simulink model "LoFT_Example3"  (R2024b)
settings: Solver=ode4  StartTime=0.0  StopTime=300  FixedStep=simu.dt  RelTol=1e-3
undefined symbols (not defined in the file): body, circtime, Communication, D1, Delta, irkb, line, LoFT, p0, Pn, s, simu, trip_time, Turbwind, waves, wind
libraries: simulink x350, spsThreePhaseVIMeasurementLib x41, spsThreePhasePISectionLineLib x34, spsThreePhaseParallelRLCLoadLib x21, spsThreePhaseTransformerTwoWindingsLib x14, spsLoadFlowBusLib x10, spsThreePhaseDynamicLoadLib x9, spsSynchronousMachinepuStandardLib x7, spsExcitationSystemLib x7, spsSteamTurbineandGovernorLib x7, spsGenericPowerSystemStabilizerLib x7, spsMultiBandPowerSystemStabilizerLib x7
(part 2 of 49)

== system LoFT_Example3/FOWT System/Subsystem13 ==
  action : Inport
  In2 : Inport  Port=2
  In1 : Inport  Port=3
  Constant1 : Constant  Value=Communication(5)
  Constant10 : Constant  Value=Communication(3)
  Constant11 : Constant  Value=Communication(9)
  Constant12 : Constant  Value=Communication(6)
  Constant14 : Constant  Value=Communication(7)
  Constant16 : Constant  Value=Communication(8)
  Constant19 : Constant  Value=Communication(10)
  Constant7 : Constant  Value=Communication(4)
  Constant8 : Constant  Value=Communication(1)
  Constant9 : Constant  Value=Communication(2)
  Demux : Demux  Outputs=10
  Demux1 : Demux  Outputs=10
  FOWT1 : Subsystem  mask{Aero=LoFT.Aero, Hydro=LoFT.Hydro, Mooring=LoFT.Mooring, Property=LoFT.Property, Controller=LoFT.Controller, Initposition=[15,  0,  3*pi/180], Initstate=[6.8*pi/30, 9]}
      mask prompts: Aero "Aerodynamics"; Hydro "Hydrodynamics"; Mooring "Mooring lookup table"; Property "Hull mass, inertia and volume"; Controller "Local controller"; Initposition "Initial Hull position"; Initstate "Initial RotSpeed and WindEst"
      mask DialogControl DescGroupVar Prompt: LoFT
      mask DialogControl FOWT Prompt: Low-order modelling of floating offshore wind turbine for training
      mask DialogControl Manuscript Prompt: Citation
      mask DialogControl scriptname Prompt: Primary Frequency Response of Floating Offshore Wind Turbines via Deep Reinforcement Learning and Domain Randomization
      mask DialogControl ParameterGroupVar Prompt: 参数
  FOWT10 : Subsystem  mask{Aero=LoFT.Aero, Hydro=LoFT.Hydro, Mooring=LoFT.Mooring, Property=LoFT.Property, Controller=LoFT.Controller, Initposition=[5,  0,  3*pi/180], Initstate=[6.8*pi/30, 9]}
      mask prompts: Aero "Aerodynamics"; Hydro "Hydrodynamics"; Mooring "Mooring lookup table"; Property "Hull mass, inertia and volume"; Controller "Local controller"; Initposition "Initial Hull position"; Initstate "Initial RotSpeed and WindEst"
      mask DialogControl DescGroupVar Prompt: LoFT
      mask DialogControl FOWT Prompt: Low-order modelling of floating offshore wind turbine for training
      mask DialogControl Manuscript Prompt: Citation
      mask DialogControl scriptname Prompt: Primary Frequency Response of Floating Offshore Wind Turbines via Deep Reinforcement Learning and Domain Randomization
      mask DialogControl ParameterGroupVar Prompt: 参数
  FOWT2 : Subsystem  mask{Aero=LoFT.Aero, Hydro=LoFT.Hydro, Mooring=LoFT.Mooring, Property=LoFT.Property, Controller=LoFT.Controller, Initposition=[40,  0,  3*pi/180], Initstate=[6.8*pi/30, 9]}
      mask prompts: Aero "Aerodynamics"; Hydro "Hydrodynamics"; Mooring "Mooring lookup table"; Property "Hull mass, inertia and volume"; Controller "Local controller"; Initposition "Initial Hull position"; Initstate "Initial RotSpeed and WindEst"
      mask DialogControl DescGroupVar Prompt: LoFT
      mask DialogControl FOWT Prompt: Low-order modelling of floating offshore wind turbine for training
      mask DialogControl Manuscript Prompt: Citation
      mask DialogControl scriptname Prompt: Primary Frequency Response of Floating Offshore Wind Turbines via Deep Reinforcement Learning and Domain Randomization
      mask DialogControl ParameterGroupVar Prompt: 参数
  FOWT3 : Subsystem  mask{Aero=LoFT.Aero, Hydro=LoFT.Hydro, Mooring=LoFT.Mooring, Property=LoFT.Property, Controller=LoFT.Controller, Initposition=[25,  0,  3*pi/180], Initstate=[6.8*pi/30, 9]}
      mask prompts: Aero "Aerodynamics"; Hydro "Hydrodynamics"; Mooring "Mooring lookup table"; Property "Hull mass, inertia and volume"; Controller "Local controller"; Initposition "Initial Hull position"; Initstate "Initial RotSpeed and WindEst"
      mask DialogControl DescGroupVar Prompt: LoFT
      mask DialogControl FOWT Prompt: Low-order modelling of floating offshore wind turbine for training
      mask DialogControl Manuscript Prompt: Citation
      mask DialogControl scriptname Prompt: Primary Frequency Response of Floating Offshore Wind Turbines via Deep Reinforcement Learning and Domain Randomization
      mask DialogControl ParameterGroupVar Prompt: 参数
  FOWT4 : Subsystem  mask{Aero=LoFT.Aero, Hydro=LoFT.Hydro, Mooring=LoFT.Mooring, Property=LoFT.Property, Controller=LoFT.Controller, Initposition=[15,  0,  3*pi/180], Initstate=[6.8*pi/30, 9]}
      mask prompts: Aero "Aerodynamics"; Hydro "Hydrodynamics"; Mooring "Mooring lookup table"; Property "Hull mass, inertia and volume"; Controller "Local controller"; Initposition "Initial Hull position"; Initstate "Initial RotSpeed and WindEst"
      mask DialogControl DescGroupVar Prompt: LoFT
      mask DialogControl FOWT Prompt: Low-order modelling of floating offshore wind turbine for training
      mask DialogControl Manuscript Prompt: Citation
      mask DialogControl scriptname Prompt: Primary Frequency Response of Floating Offshore Wind Turbines via Deep Reinforcement Learning and Domain Randomization
      mask DialogControl ParameterGroupVar Prompt: 参数
  FOWT5 : Subsystem  mask{Aero=LoFT.Aero, Hydro=LoFT.Hydro, Mooring=LoFT.Mooring, Property=LoFT.Property, Controller=LoFT.Controller, Initposition=[40,  0,  3*pi/180], Initstate=[6.8*pi/30, 9]}
      mask prompts: Aero "Aerodynamics"; Hydro "Hydrodynamics"; Mooring "Mooring lookup table"; Property "Hull mass, inertia and volume"; Controller "Local controller"; Initposition "Initial Hull position"; Initstate "Initial RotSpeed and WindEst"
      mask DialogControl DescGroupVar Prompt: LoFT
      mask DialogControl FOWT Prompt: Low-order modelling of floating offshore wind turbine for training
      mask DialogControl Manuscript Prompt: Citation
      mask DialogControl scriptname Prompt: Primary Frequency Response of Floating Offshore Wind Turbines via Deep Reinforcement Learning and Domain Randomization
      mask DialogControl ParameterGroupVar Prompt: 参数
  FOWT6 : Subsystem  mask{Aero=LoFT.Aero, Hydro=LoFT.Hydro, Mooring=LoFT.Mooring, Property=LoFT.Property, Controller=LoFT.Controller, Initposition=[25,  0,  3*pi/180], Initstate=[6.8*pi/30, 9]}
      mask prompts: Aero "Aerodynamics"; Hydro "Hydrodynamics"; Mooring "Mooring lookup table"; Property "Hull mass, inertia and volume"; Controller "Local controller"; Initposition "Initial Hull position"; Initstate "Initial RotSpeed and WindEst"
      mask DialogControl DescGroupVar Prompt: LoFT
      mask DialogControl FOWT Prompt: Low-order modelling of floating offshore wind turbine for training
      mask DialogControl Manuscript Prompt: Citation
      mask DialogControl scriptname Prompt: Primary Frequency Response of Floating Offshore Wind Turbines via Deep Reinforcement Learning and Domain Randomization
      mask DialogControl ParameterGroupVar Prompt: 参数
  FOWT7 : Subsystem  mask{Aero=LoFT.Aero, Hydro=LoFT.Hydro, Mooring=LoFT.Mooring, Property=LoFT.Property, Controller=LoFT.Controller, Initposition=[15,  0,  3*pi/180], Initstate=[6.8*pi/30, 9]}
      mask prompts: Aero "Aerodynamics"; Hydro "Hydrodynamics"; Mooring "Mooring lookup table"; Property "Hull mass, inertia and volume"; Controller "Local controller"; Initposition "Initial Hull position"; Initstate "Initial RotSpeed and WindEst"
      mask DialogControl DescGroupVar Prompt: LoFT
      mask DialogControl FOWT Prompt: Low-order modelling of floating offshore wind turbine for training
      mask DialogControl Manuscript Prompt: Citation
      mask DialogControl scriptname Prompt: Primary Frequency Response of Floating Offshore Wind Turbines via Deep Reinforcement Learning and Domain Randomization
      mask DialogControl ParameterGroupVar Prompt: 参数
  FOWT8 : Subsystem  mask{Aero=LoFT.Aero, Hydro=LoFT.Hydro, Mooring=LoFT.Mooring, Property=LoFT.Property, Controller=LoFT.Controller, Initposition=[40,  0,  3*pi/180], Initstate=[6.8*pi/30, 9]}
      mask prompts: Aero "Aerodynamics"; Hydro "Hydrodynamics"; Mooring "Mooring lookup table"; Property "Hull mass, inertia and volume"; Controller "Local controller"; Initposition "Initial Hull position"; Initstate "Initial RotSpeed and WindEst"
      mask DialogControl DescGroupVar Prompt: LoFT
      mask DialogControl FOWT Prompt: Low-order modelling of floating offshore wind turbine for training
      mask DialogControl Manuscript Prompt: Citation
      mask DialogControl scriptname Prompt: Primary Frequency Response of Floating Offshore Wind Turbines via Deep Reinforcement Learning and Domain Randomization
      mask DialogControl ParameterGroupVar Prompt: 参数
  FOWT9 : Subsystem  mask{Aero=LoFT.Aero, Hydro=LoFT.Hydro, Mooring=LoFT.Mooring, Property=LoFT.Property, Controller=LoFT.Controller, Initposition=[25,  0,  3*pi/180], Initstate=[6.8*pi/30, 9]}
      mask prompts: Aero "Aerodynamics"; Hydro "Hydrodynamics"; Mooring "Mooring lookup table"; Property "Hull mass, inertia and volume"; Controller "Local controller"; Initposition "Initial Hull position"; Initstate "Initial RotSpeed and WindEst"
      mask DialogControl DescGroupVar Prompt: LoFT
      mask DialogControl FOWT Prompt: Low-order modelling of floating offshore wind turbine for training
      mask DialogControl Manuscript Prompt: Citation
      mask DialogControl scriptname Prompt: Primary Frequency Response of Floating Offshore Wind Turbines via Deep Reinforcement Learning and Domain Randomization
      mask DialogControl ParameterGroupVar Prompt: 参数
  "switch " : Subsystem
  switch 1 : Subsystem
  switch 2 : Subsystem
  switch 3 : Subsystem
  switch 4 : Subsystem
  switch 5 : Subsystem
  switch 6 : Subsystem
  switch 7 : Subsystem
  switch 8 : Subsystem
  switch 9 : Subsystem
  wave series 1 : Subsystem
  wave series 10 : Subsystem
  wave series 2 : Subsystem
  wave series 3 : Subsystem
  wave series 4 : Subsystem
  wave series 5 : Subsystem
  wave series 6 : Subsystem
  wave series 7 : Subsystem
  wave series 8 : Subsystem
  wave series 9 : Subsystem
  1 : Outport
  2 : Outport  Port=2
  3 : Outport  Port=3
  4 : Outport  Port=4
  5 : Outport  Port=5
  6 : Outport  Port=6
  7 : Outport  Port=7
  8 : Outport  Port=8
  9 : Outport  Port=9
  10 : Outport  Port=10
  wires:
  [B1] -> FOWT6/4(Blade Pitch(rad))
  [B1] -> FOWT5/4(Blade Pitch(rad))
  [B1] -> FOWT4/4(Blade Pitch(rad))
  [B1] -> FOWT3/4(Blade Pitch(rad))
  [B1] -> FOWT2/4(Blade Pitch(rad))
  [B1] -> FOWT1/4(Blade Pitch(rad))
  In1/1 -> [B1]
  FOWT10/1(Out1) -> 10/1
  FOWT9/1(Out1) -> 9/1
  FOWT8/1(Out1) -> 8/1
  FOWT7/1(Out1) -> 7/1
  FOWT6/1(Out1) -> 6/1
  FOWT5/1(Out1) -> 5/1
  FOWT4/1(Out1) -> 4/1
  FOWT3/1(Out1) -> 3/1
  FOWT2/1(Out1) -> 2/1
  FOWT1/1(Out1) -> 1/1
  Demux1/6 -> [Wind6]
  Demux1/1 -> [Wind1]
  Demux1/10 -> [Wind10]
  Demux1/9 -> [Wind9]
  Demux1/5 -> [Wind5]
  Demux1/2 -> [Wind2]
  Demux1/3 -> [Wind3]
  Demux1/8 -> [Wind8]
  Demux1/7 -> [Wind7]
  In2/1 -> Demux1/1
  Demux1/4 -> [Wind4]
  switch 2/1(Out1) -> FOWT3/5(Commu)
  switch 3/1(Out1) -> FOWT4/5(Commu)
  switch 5/1(Out1) -> FOWT6/5(Commu)
  [P7] -> FOWT7/3(Power(MW))
  Constant9/1 -> switch 1/1(In1)
  Constant7/1 -> switch 3/1(In1)
  wave series 3/1(Out1) -> FOWT3/2(Waveforces)
  [Wind6] -> FOWT6/1(Inflow wind(m/s))
  [P2] -> FOWT2/3(Power(MW))
  [Wind1] -> FOWT1/1(Inflow wind(m/s))
  switch 1/1(Out1) -> FOWT2/5(Commu)
  Constant1/1 -> switch 4/1(In1)
  [P3] -> FOWT3/3(Power(MW))
  [B1] -> FOWT7/4(Blade Pitch(rad))
  [P1] -> FOWT1/3(Power(MW))
  [Wind7] -> FOWT7/1(Inflow wind(m/s))
  wave series 7/1(Out1) -> FOWT7/2(Waveforces)
  [P4] -> FOWT4/3(Power(MW))
  Constant12/1 -> switch 5/1(In1)
  [P6] -> FOWT6/3(Power(MW))
  Constant14/1 -> switch 6/1(In1)
  [P5] -> FOWT5/3(Power(MW))
  Constant10/1 -> switch 2/1(In1)
  wave series 5/1(Out1) -> FOWT5/2(Waveforces)
  [B1] -> FOWT8/4(Blade Pitch(rad))
  [P8] -> FOWT8/3(Power(MW))
  "switch "/1(Out1) -> FOWT1/5(Commu)
  Constant8/1 -> "switch "/1(In1)
  [Wind5] -> FOWT5/1(Inflow wind(m/s))
  wave series 1/1(Out1) -> FOWT1/2(Waveforces)
  [Wind8] -> FOWT8/1(Inflow wind(m/s))
  wave series 6/1(Out1) -> FOWT6/2(Waveforces)
  Constant16/1 -> switch 7/1(In1)
  switch 6/1(Out1) -> FOWT7/5(Commu)
  wave series 4/1(Out1) -> FOWT4/2(Waveforces)
  switch 7/1(Out1) -> FOWT8/5(Commu)
  switch 4/1(Out1) -> FOWT5/5(Commu)
  [Wind3] -> FOWT3/1(Inflow wind(m/s))
  wave series 8/1(Out1) -> FOWT8/2(Waveforces)
  [Wind4] -> FOWT4/1(Inflow wind(m/s))
  wave series 2/1(Out1) -> FOWT2/2(Waveforces)
  [Wind2] -> FOWT2/1(Inflow wind(m/s))
  Demux/2 -> [P2]
  Demux/3 -> [P3]
  action/1 -> Demux/1
  Demux/4 -> [P4]
  Demux/1 -> [P1]
  Demux/5 -> [P5]
  Demux/8 -> [P8]
  Demux/7 -> [P7]
  Demux/6 -> [P6]
  wave series 9/1(Out1) -> FOWT9/2(Waveforces)
  switch 8/1(Out1) -> FOWT9/5(Commu)
  [Wind9] -> FOWT9/1(Inflow wind(m/s))
  [B1] -> FOWT9/4(Blade Pitch(rad))
  [P9] -> FOWT9/3(Power(MW))
  Constant11/1 -> switch 8/1(In1)
  [Wind10] -> FOWT10/1(Inflow wind(m/s))
  [P10] -> FOWT10/3(Power(MW))
  switch 9/1(Out1) -> FOWT10/5(Commu)
  Constant19/1 -> switch 9/1(In1)
  [B1] -> FOWT10/4(Blade Pitch(rad))
  wave series 10/1(Out1) -> FOWT10/2(Waveforces)
  Demux/10 -> [P10]
  Demux/9 -> [P9]

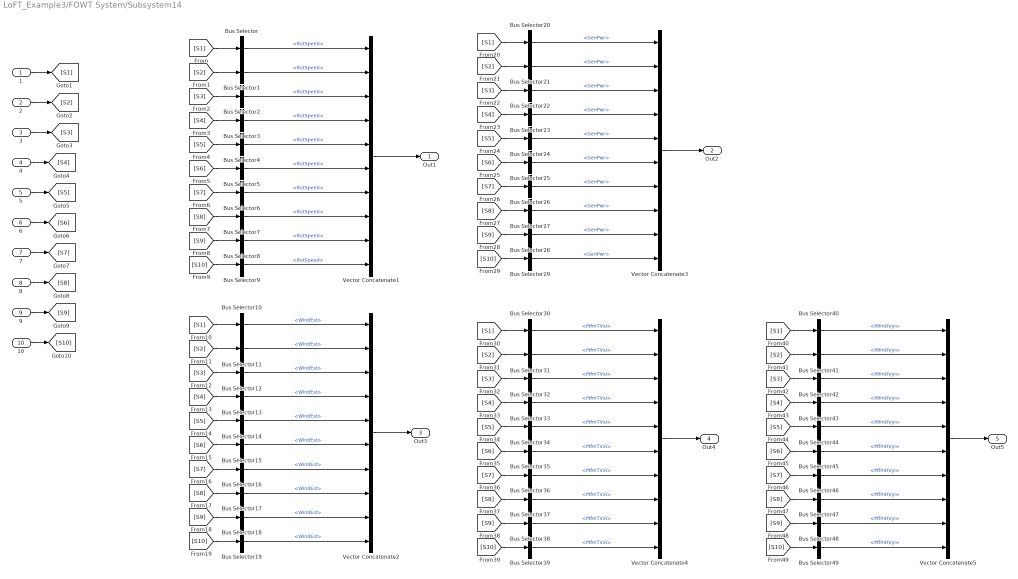
== system LoFT_Example3/FOWT System/Subsystem14 ==
  1 : Inport
  2 : Inport  Port=2
  3 : Inport  Port=3
  4 : Inport  Port=4
  5 : Inport  Port=5
  6 : Inport  Port=6
  7 : Inport  Port=7
  8 : Inport  Port=8
  9 : Inport  Port=9
  10 : Inport  Port=10
  Bus Selector{,1..9} (10 alike) : BusSelector  OutputSignals=RotSpeed
  Bus Selector{10..19} (10 alike) : BusSelector  OutputSignals=WindEst
  Bus Selector{20..29} (10 alike) : BusSelector  OutputSignals=GenPwr
  Bus Selector{30..39} (10 alike) : BusSelector  OutputSignals=PtfmTVxi
  Bus Selector{40..49} (10 alike) : BusSelector  OutputSignals=PtfmRVyi
  Vector Concatenate{1..5} (5 alike) : Concatenate  NumInputs=10
  Out1 : Outport
  Out2 : Outport  Port=2
  Out3 : Outport  Port=3
  Out4 : Outport  Port=4
  Out5 : Outport  Port=5
  wires:
  1/1 -> [S1]
  2/1 -> [S2]
  3/1 -> [S3]
  4/1 -> [S4]
  5/1 -> [S5]
  6/1 -> [S6]
  7/1 -> [S7]
  8/1 -> [S8]
  9/1 -> [S9]
  10/1 -> [S10]
  [S1] -> Bus Selector/1
  Vector Concatenate1/1 -> Out1/1
  Bus Selector/1 -> Vector Concatenate1/1  "<RotSpeed>"
  [S2] -> Bus Selector1/1
  Bus Selector1/1 -> Vector Concatenate1/2  "<RotSpeed>"
  Bus Selector2/1 -> Vector Concatenate1/3  "<RotSpeed>"
  [S3] -> Bus Selector2/1
  [S4] -> Bus Selector3/1
  Bus Selector3/1 -> Vector Concatenate1/4  "<RotSpeed>"
  [S5] -> Bus Selector4/1
  [S6] -> Bus Selector5/1
  [S7] -> Bus Selector6/1
  [S8] -> Bus Selector7/1
  [S9] -> Bus Selector8/1
  [S10] -> Bus Selector9/1
  Bus Selector4/1 -> Vector Concatenate1/5  "<RotSpeed>"
  Bus Selector5/1 -> Vector Concatenate1/6  "<RotSpeed>"
  Bus Selector6/1 -> Vector Concatenate1/7  "<RotSpeed>"
  Bus Selector7/1 -> Vector Concatenate1/8  "<RotSpeed>"
  Bus Selector8/1 -> Vector Concatenate1/9  "<RotSpeed>"
  Bus Selector9/1 -> Vector Concatenate1/10  "<RotSpeed>"
  Bus Selector19/1 -> Vector Concatenate2/10  "<WindEst>"
  Bus Selector18/1 -> Vector Concatenate2/9  "<WindEst>"
  Bus Selector17/1 -> Vector Concatenate2/8  "<WindEst>"
  Bus Selector16/1 -> Vector Concatenate2/7  "<WindEst>"
  Bus Selector15/1 -> Vector Concatenate2/6  "<WindEst>"
  Bus Selector14/1 -> Vector Concatenate2/5  "<WindEst>"
  [S10] -> Bus Selector19/1
  [S9] -> Bus Selector18/1
  [S7] -> Bus Selector16/1
  [S6] -> Bus Selector15/1
  [S5] -> Bus Selector14/1
  Bus Selector13/1 -> Vector Concatenate2/4  "<WindEst>"
  [S4] -> Bus Selector13/1
  [S3] -> Bus Selector12/1
  Bus Selector12/1 -> Vector Concatenate2/3  "<WindEst>"
  Bus Selector11/1 -> Vector Concatenate2/2  "<WindEst>"
  [S2] -> Bus Selector11/1
  Bus Selector10/1 -> Vector Concatenate2/1  "<WindEst>"
  [S1] -> Bus Selector10/1
  [S1] -> Bus Selector20/1
  Bus Selector20/1 -> Vector Concatenate3/1  "<GenPwr>"
  [S2] -> Bus Selector21/1
  Bus Selector21/1 -> Vector Concatenate3/2  "<GenPwr>"
  Bus Selector22/1 -> Vector Concatenate3/3  "<GenPwr>"
  [S3] -> Bus Selector22/1
  [S4] -> Bus Selector23/1
  Bus Selector23/1 -> Vector Concatenate3/4  "<GenPwr>"
  [S5] -> Bus Selector24/1
  [S6] -> Bus Selector25/1
  [S7] -> Bus Selector26/1
  [S8] -> Bus Selector27/1
  [S9] -> Bus Selector28/1
  [S10] -> Bus Selector29/1
  Bus Selector24/1 -> Vector Concatenate3/5  "<GenPwr>"
  Bus Selector25/1 -> Vector Concatenate3/6  "<GenPwr>"
  Bus Selector26/1 -> Vector Concatenate3/7  "<GenPwr>"
  Bus Selector27/1 -> Vector Concatenate3/8  "<GenPwr>"
  Bus Selector28/1 -> Vector Concatenate3/9  "<GenPwr>"
  Bus Selector29/1 -> Vector Concatenate3/10  "<GenPwr>"
  [S8] -> Bus Selector17/1
  Vector Concatenate3/1 -> Out2/1
  Vector Concatenate2/1 -> Out3/1
  [S1] -> Bus Selector30/1
  Bus Selector30/1 -> Vector Concatenate4/1  "<PtfmTVxi>"
  Vector Concatenate4/1 -> Out4/1
  [S5] -> Bus Selector44/1
  Bus Selector47/1 -> Vector Concatenate5/8  "<PtfmRVyi>"
  [S1] -> Bus Selector40/1
  Bus Selector40/1 -> Vector Concatenate5/1  "<PtfmRVyi>"
  [S2] -> Bus Selector41/1
  [S4] -> Bus Selector43/1
  [S3] -> Bus Selector42/1
  Bus Selector42/1 -> Vector Concatenate5/3  "<PtfmRVyi>"
  Bus Selector44/1 -> Vector Concatenate5/5  "<PtfmRVyi>"
  Bus Selector43/1 -> Vector Concatenate5/4  "<PtfmRVyi>"
  [S9] -> Bus Selector48/1
  Bus Selector45/1 -> Vector Concatenate5/6  "<PtfmRVyi>"
  Bus Selector48/1 -> Vector Concatenate5/9  "<PtfmRVyi>"
  [S6] -> Bus Selector45/1
  [S10] -> Bus Selector49/1
  Bus Selector49/1 -> Vector Concatenate5/10  "<PtfmRVyi>"
  Vector Concatenate5/1 -> Out5/1
  [S7] -> Bus Selector46/1
  Bus Selector46/1 -> Vector Concatenate5/7  "<PtfmRVyi>"
  Bus Selector41/1 -> Vector Concatenate5/2  "<PtfmRVyi>"
  [S8] -> Bus Selector47/1
  Bus Selector31/1 -> Vector Concatenate4/2  "<PtfmTVxi>"
  [S2] -> Bus Selector31/1
  Bus Selector32/1 -> Vector Concatenate4/3  "<PtfmTVxi>"
  [S3] -> Bus Selector32/1
  [S4] -> Bus Selector33/1
  Bus Selector33/1 -> Vector Concatenate4/4  "<PtfmTVxi>"
  [S5] -> Bus Selector34/1
  Bus Selector34/1 -> Vector Concatenate4/5  "<PtfmTVxi>"
  [S6] -> Bus Selector35/1
  Bus Selector35/1 -> Vector Concatenate4/6  "<PtfmTVxi>"
  [S7] -> Bus Selector36/1
  Bus Selector36/1 -> Vector Concatenate4/7  "<PtfmTVxi>"
  [S8] -> Bus Selector37/1
  Bus Selector37/1 -> Vector Concatenate4/8  "<PtfmTVxi>"
  [S9] -> Bus Selector38/1
  Bus Selector38/1 -> Vector Concatenate4/9  "<PtfmTVxi>"
  [S10] -> Bus Selector39/1
  Bus Selector39/1 -> Vector Concatenate4/10  "<PtfmTVxi>"

== system LoFT_Example3/FOWT System/Subsystem2 ==
  action : Inport
  In2 : Inport  Port=2
  In1 : Inport  Port=3
  Constant1 : Constant  Value=Communication(5)
  Constant10 : Constant  Value=Communication(3)
  Constant11 : Constant  Value=Communication(9)
  Constant12 : Constant  Value=Communication(6)
  Constant14 : Constant  Value=Communication(7)
  Constant16 : Constant  Value=Communication(8)
  Constant19 : Constant  Value=Communication(10)
  Constant7 : Constant  Value=Communication(4)
  Constant8 : Constant  Value=Communication(1)
  Constant9 : Constant  Value=Communication(2)
  Demux : Demux  Outputs=10
  Demux1 : Demux  Outputs=10
  FOWT1 : Subsystem  mask{Aero=LoFT.Aero, Hydro=LoFT.Hydro, Mooring=LoFT.Mooring, Property=LoFT.Property, Controller=LoFT.Controller, Initposition=[15,  0,  3*pi/180], Initstate=[6.8*pi/30, 9]}
      mask prompts: Aero "Aerodynamics"; Hydro "Hydrodynamics"; Mooring "Mooring lookup table"; Property "Hull mass, inertia and volume"; Controller "Local controller"; Initposition "Initial Hull position"; Initstate "Initial RotSpeed and WindEst"
      mask DialogControl DescGroupVar Prompt: LoFT
      mask DialogControl FOWT Prompt: Low-order modelling of floating offshore wind turbine for training
      mask DialogControl Manuscript Prompt: Citation
      mask DialogControl scriptname Prompt: Primary Frequency Response of Floating Offshore Wind Turbines via Deep Reinforcement Learning and Domain Randomization
      mask DialogControl ParameterGroupVar Prompt: 参数
  FOWT10 : Subsystem  mask{Aero=LoFT.Aero, Hydro=LoFT.Hydro, Mooring=LoFT.Mooring, Property=LoFT.Property, Controller=LoFT.Controller, Initposition=[5,  0,  3*pi/180], Initstate=[6.8*pi/30, 9]}
      mask prompts: Aero "Aerodynamics"; Hydro "Hydrodynamics"; Mooring "Mooring lookup table"; Property "Hull mass, inertia and volume"; Controller "Local controller"; Initposition "Initial Hull position"; Initstate "Initial RotSpeed and WindEst"
      mask DialogControl DescGroupVar Prompt: LoFT
      mask DialogControl FOWT Prompt: Low-order modelling of floating offshore wind turbine for training
      mask DialogControl Manuscript Prompt: Citation
      mask DialogControl scriptname Prompt: Primary Frequency Response of Floating Offshore Wind Turbines via Deep Reinforcement Learning and Domain Randomization
      mask DialogControl ParameterGroupVar Prompt: 参数
  FOWT2 : Subsystem  mask{Aero=LoFT.Aero, Hydro=LoFT.Hydro, Mooring=LoFT.Mooring, Property=LoFT.Property, Controller=LoFT.Controller, Initposition=[40,  0,  3*pi/180], Initstate=[6.8*pi/30, 9]}
      mask prompts: Aero "Aerodynamics"; Hydro "Hydrodynamics"; Mooring "Mooring lookup table"; Property "Hull mass, inertia and volume"; Controller "Local controller"; Initposition "Initial Hull position"; Initstate "Initial RotSpeed and WindEst"
      mask DialogControl DescGroupVar Prompt: LoFT
      mask DialogControl FOWT Prompt: Low-order modelling of floating offshore wind turbine for training
      mask DialogControl Manuscript Prompt: Citation
      mask DialogControl scriptname Prompt: Primary Frequency Response of Floating Offshore Wind Turbines via Deep Reinforcement Learning and Domain Randomization
      mask DialogControl ParameterGroupVar Prompt: 参数
  FOWT3 : Subsystem  mask{Aero=LoFT.Aero, Hydro=LoFT.Hydro, Mooring=LoFT.Mooring, Property=LoFT.Property, Controller=LoFT.Controller, Initposition=[25,  0,  3*pi/180], Initstate=[6.8*pi/30, 9]}
      mask prompts: Aero "Aerodynamics"; Hydro "Hydrodynamics"; Mooring "Mooring lookup table"; Property "Hull mass, inertia and volume"; Controller "Local controller"; Initposition "Initial Hull position"; Initstate "Initial RotSpeed and WindEst"
      mask DialogControl DescGroupVar Prompt: LoFT
      mask DialogControl FOWT Prompt: Low-order modelling of floating offshore wind turbine for training
      mask DialogControl Manuscript Prompt: Citation
      mask DialogControl scriptname Prompt: Primary Frequency Response of Floating Offshore Wind Turbines via Deep Reinforcement Learning and Domain Randomization
      mask DialogControl ParameterGroupVar Prompt: 参数
  FOWT4 : Subsystem  mask{Aero=LoFT.Aero, Hydro=LoFT.Hydro, Mooring=LoFT.Mooring, Property=LoFT.Property, Controller=LoFT.Controller, Initposition=[15,  0,  3*pi/180], Initstate=[6.8*pi/30, 9]}
      mask prompts: Aero "Aerodynamics"; Hydro "Hydrodynamics"; Mooring "Mooring lookup table"; Property "Hull mass, inertia and volume"; Controller "Local controller"; Initposition "Initial Hull position"; Initstate "Initial RotSpeed and WindEst"
      mask DialogControl DescGroupVar Prompt: LoFT
      mask DialogControl FOWT Prompt: Low-order modelling of floating offshore wind turbine for training
      mask DialogControl Manuscript Prompt: Citation
      mask DialogControl scriptname Prompt: Primary Frequency Response of Floating Offshore Wind Turbines via Deep Reinforcement Learning and Domain Randomization
      mask DialogControl ParameterGroupVar Prompt: 参数
  FOWT5 : Subsystem  mask{Aero=LoFT.Aero, Hydro=LoFT.Hydro, Mooring=LoFT.Mooring, Property=LoFT.Property, Controller=LoFT.Controller, Initposition=[40,  0,  3*pi/180], Initstate=[6.8*pi/30, 9]}
      mask prompts: Aero "Aerodynamics"; Hydro "Hydrodynamics"; Mooring "Mooring lookup table"; Property "Hull mass, inertia and volume"; Controller "Local controller"; Initposition "Initial Hull position"; Initstate "Initial RotSpeed and WindEst"
      mask DialogControl DescGroupVar Prompt: LoFT
      mask DialogControl FOWT Prompt: Low-order modelling of floating offshore wind turbine for training
      mask DialogControl Manuscript Prompt: Citation
      mask DialogControl scriptname Prompt: Primary Frequency Response of Floating Offshore Wind Turbines via Deep Reinforcement Learning and Domain Randomization
      mask DialogControl ParameterGroupVar Prompt: 参数
  FOWT6 : Subsystem  mask{Aero=LoFT.Aero, Hydro=LoFT.Hydro, Mooring=LoFT.Mooring, Property=LoFT.Property, Controller=LoFT.Controller, Initposition=[25,  0,  3*pi/180], Initstate=[6.8*pi/30, 9]}
      mask prompts: Aero "Aerodynamics"; Hydro "Hydrodynamics"; Mooring "Mooring lookup table"; Property "Hull mass, inertia and volume"; Controller "Local controller"; Initposition "Initial Hull position"; Initstate "Initial RotSpeed and WindEst"
      mask DialogControl DescGroupVar Prompt: LoFT
      mask DialogControl FOWT Prompt: Low-order modelling of floating offshore wind turbine for training
      mask DialogControl Manuscript Prompt: Citation
      mask DialogControl scriptname Prompt: Primary Frequency Response of Floating Offshore Wind Turbines via Deep Reinforcement Learning and Domain Randomization
      mask DialogControl ParameterGroupVar Prompt: 参数
  FOWT7 : Subsystem  mask{Aero=LoFT.Aero, Hydro=LoFT.Hydro, Mooring=LoFT.Mooring, Property=LoFT.Property, Controller=LoFT.Controller, Initposition=[15,  0,  3*pi/180], Initstate=[6.8*pi/30, 9]}
      mask prompts: Aero "Aerodynamics"; Hydro "Hydrodynamics"; Mooring "Mooring lookup table"; Property "Hull mass, inertia and volume"; Controller "Local controller"; Initposition "Initial Hull position"; Initstate "Initial RotSpeed and WindEst"
      mask DialogControl DescGroupVar Prompt: LoFT
      mask DialogControl FOWT Prompt: Low-order modelling of floating offshore wind turbine for training
      mask DialogControl Manuscript Prompt: Citation
      mask DialogControl scriptname Prompt: Primary Frequency Response of Floating Offshore Wind Turbines via Deep Reinforcement Learning and Domain Randomization
      mask DialogControl ParameterGroupVar Prompt: 参数
  FOWT8 : Subsystem  mask{Aero=LoFT.Aero, Hydro=LoFT.Hydro, Mooring=LoFT.Mooring, Property=LoFT.Property, Controller=LoFT.Controller, Initposition=[40,  0,  3*pi/180], Initstate=[6.8*pi/30, 9]}
      mask prompts: Aero "Aerodynamics"; Hydro "Hydrodynamics"; Mooring "Mooring lookup table"; Property "Hull mass, inertia and volume"; Controller "Local controller"; Initposition "Initial Hull position"; Initstate "Initial RotSpeed and WindEst"
      mask DialogControl DescGroupVar Prompt: LoFT
      mask DialogControl FOWT Prompt: Low-order modelling of floating offshore wind turbine for training
      mask DialogControl Manuscript Prompt: Citation
      mask DialogControl scriptname Prompt: Primary Frequency Response of Floating Offshore Wind Turbines via Deep Reinforcement Learning and Domain Randomization
      mask DialogControl ParameterGroupVar Prompt: 参数
  FOWT9 : Subsystem  mask{Aero=LoFT.Aero, Hydro=LoFT.Hydro, Mooring=LoFT.Mooring, Property=LoFT.Property, Controller=LoFT.Controller, Initposition=[25,  0,  3*pi/180], Initstate=[6.8*pi/30, 9]}
      mask prompts: Aero "Aerodynamics"; Hydro "Hydrodynamics"; Mooring "Mooring lookup table"; Property "Hull mass, inertia and volume"; Controller "Local controller"; Initposition "Initial Hull position"; Initstate "Initial RotSpeed and WindEst"
      mask DialogControl DescGroupVar Prompt: LoFT
      mask DialogControl FOWT Prompt: Low-order modelling of floating offshore wind turbine for training
      mask DialogControl Manuscript Prompt: Citation
      mask DialogControl scriptname Prompt: Primary Frequency Response of Floating Offshore Wind Turbines via Deep Reinforcement Learning and Domain Randomization
      mask DialogControl ParameterGroupVar Prompt: 参数
  "switch " : Subsystem
  switch 1 : Subsystem
  switch 2 : Subsystem
  switch 3 : Subsystem
  switch 4 : Subsystem
  switch 5 : Subsystem
  switch 6 : Subsystem
  switch 7 : Subsystem
  switch 8 : Subsystem
  switch 9 : Subsystem
  wave series 1 : Subsystem
  wave series 10 : Subsystem
  wave series 2 : Subsystem
  wave series 3 : Subsystem
  wave series 4 : Subsystem
  wave series 5 : Subsystem
  wave series 6 : Subsystem
  wave series 7 : Subsystem
  wave series 8 : Subsystem
  wave series 9 : Subsystem
  1 : Outport
  2 : Outport  Port=2
  3 : Outport  Port=3
  4 : Outport  Port=4
  5 : Outport  Port=5
  6 : Outport  Port=6
  7 : Outport  Port=7
  8 : Outport  Port=8
  9 : Outport  Port=9
  10 : Outport  Port=10
  wires:
  [B1] -> FOWT6/4(Blade Pitch(rad))
  [B1] -> FOWT5/4(Blade Pitch(rad))
  [B1] -> FOWT4/4(Blade Pitch(rad))
  [B1] -> FOWT3/4(Blade Pitch(rad))
  [B1] -> FOWT2/4(Blade Pitch(rad))
  [B1] -> FOWT1/4(Blade Pitch(rad))
  In1/1 -> [B1]
  FOWT10/1(Out1) -> 10/1
  FOWT9/1(Out1) -> 9/1
  FOWT8/1(Out1) -> 8/1
  FOWT7/1(Out1) -> 7/1
  FOWT6/1(Out1) -> 6/1
  FOWT5/1(Out1) -> 5/1
  FOWT4/1(Out1) -> 4/1
  FOWT3/1(Out1) -> 3/1
  FOWT2/1(Out1) -> 2/1
  FOWT1/1(Out1) -> 1/1
  Demux1/6 -> [Wind6]
  Demux1/1 -> [Wind1]
  Demux1/10 -> [Wind10]
  Demux1/9 -> [Wind9]
  Demux1/5 -> [Wind5]
  Demux1/2 -> [Wind2]
  Demux1/3 -> [Wind3]
  Demux1/8 -> [Wind8]
  Demux1/7 -> [Wind7]
  In2/1 -> Demux1/1
  Demux1/4 -> [Wind4]
  switch 2/1(Out1) -> FOWT3/5(Commu)
  switch 3/1(Out1) -> FOWT4/5(Commu)
  switch 5/1(Out1) -> FOWT6/5(Commu)
  [P7] -> FOWT7/3(Power(MW))
  Constant9/1 -> switch 1/1(In1)
  Constant7/1 -> switch 3/1(In1)
  wave series 3/1(Out1) -> FOWT3/2(Waveforces)
  [Wind6] -> FOWT6/1(Inflow wind(m/s))
  [P2] -> FOWT2/3(Power(MW))
  [Wind1] -> FOWT1/1(Inflow wind(m/s))
  switch 1/1(Out1) -> FOWT2/5(Commu)
  Constant1/1 -> switch 4/1(In1)
  [P3] -> FOWT3/3(Power(MW))
  [B1] -> FOWT7/4(Blade Pitch(rad))
  [P1] -> FOWT1/3(Power(MW))
  [Wind7] -> FOWT7/1(Inflow wind(m/s))
  wave series 7/1(Out1) -> FOWT7/2(Waveforces)
  [P4] -> FOWT4/3(Power(MW))
  Constant12/1 -> switch 5/1(In1)
  [P6] -> FOWT6/3(Power(MW))
  Constant14/1 -> switch 6/1(In1)
  [P5] -> FOWT5/3(Power(MW))
  Constant10/1 -> switch 2/1(In1)
  wave series 5/1(Out1) -> FOWT5/2(Waveforces)
  [B1] -> FOWT8/4(Blade Pitch(rad))
  [P8] -> FOWT8/3(Power(MW))
  "switch "/1(Out1) -> FOWT1/5(Commu)
  Constant8/1 -> "switch "/1(In1)
  [Wind5] -> FOWT5/1(Inflow wind(m/s))
  wave series 1/1(Out1) -> FOWT1/2(Waveforces)
  [Wind8] -> FOWT8/1(Inflow wind(m/s))
  wave series 6/1(Out1) -> FOWT6/2(Waveforces)
  Constant16/1 -> switch 7/1(In1)
  switch 6/1(Out1) -> FOWT7/5(Commu)
  wave series 4/1(Out1) -> FOWT4/2(Waveforces)
  switch 7/1(Out1) -> FOWT8/5(Commu)
  switch 4/1(Out1) -> FOWT5/5(Commu)
  [Wind3] -> FOWT3/1(Inflow wind(m/s))
  wave series 8/1(Out1) -> FOWT8/2(Waveforces)
  [Wind4] -> FOWT4/1(Inflow wind(m/s))
  wave series 2/1(Out1) -> FOWT2/2(Waveforces)
  [Wind2] -> FOWT2/1(Inflow wind(m/s))
  Demux/2 -> [P2]
  Demux/3 -> [P3]
  action/1 -> Demux/1
  Demux/4 -> [P4]
  Demux/1 -> [P1]
  Demux/5 -> [P5]
  Demux/8 -> [P8]
  Demux/7 -> [P7]
  Demux/6 -> [P6]
  wave series 9/1(Out1) -> FOWT9/2(Waveforces)
  switch 8/1(Out1) -> FOWT9/5(Commu)
  [Wind9] -> FOWT9/1(Inflow wind(m/s))
  [B1] -> FOWT9/4(Blade Pitch(rad))
  [P9] -> FOWT9/3(Power(MW))
  Constant11/1 -> switch 8/1(In1)
  [Wind10] -> FOWT10/1(Inflow wind(m/s))
  [P10] -> FOWT10/3(Power(MW))
  switch 9/1(Out1) -> FOWT10/5(Commu)
  Constant19/1 -> switch 9/1(In1)
  [B1] -> FOWT10/4(Blade Pitch(rad))
  wave series 10/1(Out1) -> FOWT10/2(Waveforces)
  Demux/10 -> [P10]
  Demux/9 -> [P9]

== system LoFT_Example3/FOWT System/Subsystem3 ==
  action : Inport
  In2 : Inport  Port=2
  In1 : Inport  Port=3
  Constant1 : Constant  Value=Communication(5)
  Constant10 : Constant  Value=Communication(3)
  Constant11 : Constant  Value=Communication(9)
  Constant12 : Constant  Value=Communication(6)
  Constant14 : Constant  Value=Communication(7)
  Constant16 : Constant  Value=Communication(8)
  Constant19 : Constant  Value=Communication(10)
  Constant7 : Constant  Value=Communication(4)
  Constant8 : Constant  Value=Communication(1)
  Constant9 : Constant  Value=Communication(2)
  Demux : Demux  Outputs=10
  Demux1 : Demux  Outputs=10
  FOWT1 : Subsystem  mask{Aero=LoFT.Aero, Hydro=LoFT.Hydro, Mooring=LoFT.Mooring, Property=LoFT.Property, Controller=LoFT.Controller, Initposition=[15,  0,  3*pi/180], Initstate=[6.8*pi/30, 9]}
      mask prompts: Aero "Aerodynamics"; Hydro "Hydrodynamics"; Mooring "Mooring lookup table"; Property "Hull mass, inertia and volume"; Controller "Local controller"; Initposition "Initial Hull position"; Initstate "Initial RotSpeed and WindEst"
      mask DialogControl DescGroupVar Prompt: LoFT
      mask DialogControl FOWT Prompt: Low-order modelling of floating offshore wind turbine for training
      mask DialogControl Manuscript Prompt: Citation
      mask DialogControl scriptname Prompt: Primary Frequency Response of Floating Offshore Wind Turbines via Deep Reinforcement Learning and Domain Randomization
      mask DialogControl ParameterGroupVar Prompt: 参数
  FOWT10 : Subsystem  mask{Aero=LoFT.Aero, Hydro=LoFT.Hydro, Mooring=LoFT.Mooring, Property=LoFT.Property, Controller=LoFT.Controller, Initposition=[5,  0,  3*pi/180], Initstate=[6.8*pi/30, 9]}
      mask prompts: Aero "Aerodynamics"; Hydro "Hydrodynamics"; Mooring "Mooring lookup table"; Property "Hull mass, inertia and volume"; Controller "Local controller"; Initposition "Initial Hull position"; Initstate "Initial RotSpeed and WindEst"
      mask DialogControl DescGroupVar Prompt: LoFT
      mask DialogControl FOWT Prompt: Low-order modelling of floating offshore wind turbine for training
      mask DialogControl Manuscript Prompt: Citation
      mask DialogControl scriptname Prompt: Primary Frequency Response of Floating Offshore Wind Turbines via Deep Reinforcement Learning and Domain Randomization
      mask DialogControl ParameterGroupVar Prompt: 参数
  FOWT2 : Subsystem  mask{Aero=LoFT.Aero, Hydro=LoFT.Hydro, Mooring=LoFT.Mooring, Property=LoFT.Property, Controller=LoFT.Controller, Initposition=[40,  0,  3*pi/180], Initstate=[6.8*pi/30, 9]}
      mask prompts: Aero "Aerodynamics"; Hydro "Hydrodynamics"; Mooring "Mooring lookup table"; Property "Hull mass, inertia and volume"; Controller "Local controller"; Initposition "Initial Hull position"; Initstate "Initial RotSpeed and WindEst"
      mask DialogControl DescGroupVar Prompt: LoFT
      mask DialogControl FOWT Prompt: Low-order modelling of floating offshore wind turbine for training
      mask DialogControl Manuscript Prompt: Citation
      mask DialogControl scriptname Prompt: Primary Frequency Response of Floating Offshore Wind Turbines via Deep Reinforcement Learning and Domain Randomization
      mask DialogControl ParameterGroupVar Prompt: 参数
  FOWT3 : Subsystem  mask{Aero=LoFT.Aero, Hydro=LoFT.Hydro, Mooring=LoFT.Mooring, Property=LoFT.Property, Controller=LoFT.Controller, Initposition=[25,  0,  3*pi/180], Initstate=[6.8*pi/30, 9]}
      mask prompts: Aero "Aerodynamics"; Hydro "Hydrodynamics"; Mooring "Mooring lookup table"; Property "Hull mass, inertia and volume"; Controller "Local controller"; Initposition "Initial Hull position"; Initstate "Initial RotSpeed and WindEst"
      mask DialogControl DescGroupVar Prompt: LoFT
      mask DialogControl FOWT Prompt: Low-order modelling of floating offshore wind turbine for training
      mask DialogControl Manuscript Prompt: Citation
      mask DialogControl scriptname Prompt: Primary Frequency Response of Floating Offshore Wind Turbines via Deep Reinforcement Learning and Domain Randomization
      mask DialogControl ParameterGroupVar Prompt: 参数
  FOWT4 : Subsystem  mask{Aero=LoFT.Aero, Hydro=LoFT.Hydro, Mooring=LoFT.Mooring, Property=LoFT.Property, Controller=LoFT.Controller, Initposition=[15,  0,  3*pi/180], Initstate=[6.8*pi/30, 9]}
      mask prompts: Aero "Aerodynamics"; Hydro "Hydrodynamics"; Mooring "Mooring lookup table"; Property "Hull mass, inertia and volume"; Controller "Local controller"; Initposition "Initial Hull position"; Initstate "Initial RotSpeed and WindEst"
      mask DialogControl DescGroupVar Prompt: LoFT
      mask DialogControl FOWT Prompt: Low-order modelling of floating offshore wind turbine for training
      mask DialogControl Manuscript Prompt: Citation
      mask DialogControl scriptname Prompt: Primary Frequency Response of Floating Offshore Wind Turbines via Deep Reinforcement Learning and Domain Randomization
      mask DialogControl ParameterGroupVar Prompt: 参数
  FOWT5 : Subsystem  mask{Aero=LoFT.Aero, Hydro=LoFT.Hydro, Mooring=LoFT.Mooring, Property=LoFT.Property, Controller=LoFT.Controller, Initposition=[40,  0,  3*pi/180], Initstate=[6.8*pi/30, 9]}
      mask prompts: Aero "Aerodynamics"; Hydro "Hydrodynamics"; Mooring "Mooring lookup table"; Property "Hull mass, inertia and volume"; Controller "Local controller"; Initposition "Initial Hull position"; Initstate "Initial RotSpeed and WindEst"
      mask DialogControl DescGroupVar Prompt: LoFT
      mask DialogControl FOWT Prompt: Low-order modelling of floating offshore wind turbine for training
      mask DialogControl Manuscript Prompt: Citation
      mask DialogControl scriptname Prompt: Primary Frequency Response of Floating Offshore Wind Turbines via Deep Reinforcement Learning and Domain Randomization
      mask DialogControl ParameterGroupVar Prompt: 参数
  FOWT6 : Subsystem  mask{Aero=LoFT.Aero, Hydro=LoFT.Hydro, Mooring=LoFT.Mooring, Property=LoFT.Property, Controller=LoFT.Controller, Initposition=[25,  0,  3*pi/180], Initstate=[6.8*pi/30, 9]}
      mask prompts: Aero "Aerodynamics"; Hydro "Hydrodynamics"; Mooring "Mooring lookup table"; Property "Hull mass, inertia and volume"; Controller "Local controller"; Initposition "Initial Hull position"; Initstate "Initial RotSpeed and WindEst"
      mask DialogControl DescGroupVar Prompt: LoFT
      mask DialogControl FOWT Prompt: Low-order modelling of floating offshore wind turbine for training
      mask DialogControl Manuscript Prompt: Citation
      mask DialogControl scriptname Prompt: Primary Frequency Response of Floating Offshore Wind Turbines via Deep Reinforcement Learning and Domain Randomization
      mask DialogControl ParameterGroupVar Prompt: 参数
  FOWT7 : Subsystem  mask{Aero=LoFT.Aero, Hydro=LoFT.Hydro, Mooring=LoFT.Mooring, Property=LoFT.Property, Controller=LoFT.Controller, Initposition=[15,  0,  3*pi/180], Initstate=[6.8*pi/30, 9]}
      mask prompts: Aero "Aerodynamics"; Hydro "Hydrodynamics"; Mooring "Mooring lookup table"; Property "Hull mass, inertia and volume"; Controller "Local controller"; Initposition "Initial Hull position"; Initstate "Initial RotSpeed and WindEst"
      mask DialogControl DescGroupVar Prompt: LoFT
      mask DialogControl FOWT Prompt: Low-order modelling of floating offshore wind turbine for training
      mask DialogControl Manuscript Prompt: Citation
      mask DialogControl scriptname Prompt: Primary Frequency Response of Floating Offshore Wind Turbines via Deep Reinforcement Learning and Domain Randomization
      mask DialogControl ParameterGroupVar Prompt: 参数
  FOWT8 : Subsystem  mask{Aero=LoFT.Aero, Hydro=LoFT.Hydro, Mooring=LoFT.Mooring, Property=LoFT.Property, Controller=LoFT.Controller, Initposition=[40,  0,  3*pi/180], Initstate=[6.8*pi/30, 9]}
      mask prompts: Aero "Aerodynamics"; Hydro "Hydrodynamics"; Mooring "Mooring lookup table"; Property "Hull mass, inertia and volume"; Controller "Local controller"; Initposition "Initial Hull position"; Initstate "Initial RotSpeed and WindEst"
      mask DialogControl DescGroupVar Prompt: LoFT
      mask DialogControl FOWT Prompt: Low-order modelling of floating offshore wind turbine for training
      mask DialogControl Manuscript Prompt: Citation
      mask DialogControl scriptname Prompt: Primary Frequency Response of Floating Offshore Wind Turbines via Deep Reinforcement Learning and Domain Randomization
      mask DialogControl ParameterGroupVar Prompt: 参数
  FOWT9 : Subsystem  mask{Aero=LoFT.Aero, Hydro=LoFT.Hydro, Mooring=LoFT.Mooring, Property=LoFT.Property, Controller=LoFT.Controller, Initposition=[25,  0,  3*pi/180], Initstate=[6.8*pi/30, 9]}
      mask prompts: Aero "Aerodynamics"; Hydro "Hydrodynamics"; Mooring "Mooring lookup table"; Property "Hull mass, inertia and volume"; Controller "Local controller"; Initposition "Initial Hull position"; Initstate "Initial RotSpeed and WindEst"
      mask DialogControl DescGroupVar Prompt: LoFT
      mask DialogControl FOWT Prompt: Low-order modelling of floating offshore wind turbine for training
      mask DialogControl Manuscript Prompt: Citation
      mask DialogControl scriptname Prompt: Primary Frequency Response of Floating Offshore Wind Turbines via Deep Reinforcement Learning and Domain Randomization
      mask DialogControl ParameterGroupVar Prompt: 参数
  "switch " : Subsystem
  switch 1 : Subsystem
  switch 2 : Subsystem
  switch 3 : Subsystem
  switch 4 : Subsystem
  switch 5 : Subsystem
  switch 6 : Subsystem
  switch 7 : Subsystem
  switch 8 : Subsystem
  switch 9 : Subsystem
  wave series 1 : Subsystem
  wave series 10 : Subsystem
  wave series 2 : Subsystem
  wave series 3 : Subsystem
  wave series 4 : Subsystem
  wave series 5 : Subsystem
  wave series 6 : Subsystem
  wave series 7 : Subsystem
  wave series 8 : Subsystem
  wave series 9 : Subsystem
  1 : Outport
  2 : Outport  Port=2
  3 : Outport  Port=3
  4 : Outport  Port=4
  5 : Outport  Port=5
  6 : Outport  Port=6
  7 : Outport  Port=7
  8 : Outport  Port=8
  9 : Outport  Port=9
  10 : Outport  Port=10
  wires:
  Demux/9 -> [P9]
  Demux/10 -> [P10]
  wave series 10/1(Out1) -> FOWT10/2(Waveforces)
  [B1] -> FOWT10/4(Blade Pitch(rad))
  Constant19/1 -> switch 9/1(In1)
  switch 9/1(Out1) -> FOWT10/5(Commu)
  [P10] -> FOWT10/3(Power(MW))
  [Wind10] -> FOWT10/1(Inflow wind(m/s))
  Constant11/1 -> switch 8/1(In1)
  [P9] -> FOWT9/3(Power(MW))
  [B1] -> FOWT9/4(Blade Pitch(rad))
  [Wind9] -> FOWT9/1(Inflow wind(m/s))
  switch 8/1(Out1) -> FOWT9/5(Commu)
  wave series 9/1(Out1) -> FOWT9/2(Waveforces)
  Demux/6 -> [P6]
  Demux/7 -> [P7]
  Demux/8 -> [P8]
  Demux/5 -> [P5]
  Demux/1 -> [P1]
  Demux/4 -> [P4]
  action/1 -> Demux/1
  Demux/3 -> [P3]
  Demux/2 -> [P2]
  [Wind2] -> FOWT2/1(Inflow wind(m/s))
  wave series 2/1(Out1) -> FOWT2/2(Waveforces)
  [Wind4] -> FOWT4/1(Inflow wind(m/s))
  wave series 8/1(Out1) -> FOWT8/2(Waveforces)
  [Wind3] -> FOWT3/1(Inflow wind(m/s))
  switch 4/1(Out1) -> FOWT5/5(Commu)
  switch 7/1(Out1) -> FOWT8/5(Commu)
  wave series 4/1(Out1) -> FOWT4/2(Waveforces)
  switch 6/1(Out1) -> FOWT7/5(Commu)
  Constant16/1 -> switch 7/1(In1)
  wave series 6/1(Out1) -> FOWT6/2(Waveforces)
  [Wind8] -> FOWT8/1(Inflow wind(m/s))
  wave series 1/1(Out1) -> FOWT1/2(Waveforces)
  [Wind5] -> FOWT5/1(Inflow wind(m/s))
  Constant8/1 -> "switch "/1(In1)
  "switch "/1(Out1) -> FOWT1/5(Commu)
  [P8] -> FOWT8/3(Power(MW))
  [B1] -> FOWT8/4(Blade Pitch(rad))
  wave series 5/1(Out1) -> FOWT5/2(Waveforces)
  Constant10/1 -> switch 2/1(In1)
  [P5] -> FOWT5/3(Power(MW))
  Constant14/1 -> switch 6/1(In1)
  [P6] -> FOWT6/3(Power(MW))
  Constant12/1 -> switch 5/1(In1)
  [P4] -> FOWT4/3(Power(MW))
  wave series 7/1(Out1) -> FOWT7/2(Waveforces)
  [Wind7] -> FOWT7/1(Inflow wind(m/s))
  [P1] -> FOWT1/3(Power(MW))
  [B1] -> FOWT7/4(Blade Pitch(rad))
  [P3] -> FOWT3/3(Power(MW))
  Constant1/1 -> switch 4/1(In1)
  switch 1/1(Out1) -> FOWT2/5(Commu)
  [Wind1] -> FOWT1/1(Inflow wind(m/s))
  [P2] -> FOWT2/3(Power(MW))
  [Wind6] -> FOWT6/1(Inflow wind(m/s))
  wave series 3/1(Out1) -> FOWT3/2(Waveforces)
  Constant7/1 -> switch 3/1(In1)
  Constant9/1 -> switch 1/1(In1)
  [P7] -> FOWT7/3(Power(MW))
  switch 5/1(Out1) -> FOWT6/5(Commu)
  switch 3/1(Out1) -> FOWT4/5(Commu)
  switch 2/1(Out1) -> FOWT3/5(Commu)
  Demux1/4 -> [Wind4]
  In2/1 -> Demux1/1
  Demux1/7 -> [Wind7]
  Demux1/8 -> [Wind8]
  Demux1/3 -> [Wind3]
  Demux1/2 -> [Wind2]
  Demux1/5 -> [Wind5]
  Demux1/9 -> [Wind9]
  Demux1/10 -> [Wind10]
  Demux1/1 -> [Wind1]
  Demux1/6 -> [Wind6]
  FOWT1/1(Out1) -> 1/1
  FOWT2/1(Out1) -> 2/1
  FOWT3/1(Out1) -> 3/1
  FOWT4/1(Out1) -> 4/1
  FOWT5/1(Out1) -> 5/1
  FOWT6/1(Out1) -> 6/1
  FOWT7/1(Out1) -> 7/1
  FOWT8/1(Out1) -> 8/1
  FOWT9/1(Out1) -> 9/1
  FOWT10/1(Out1) -> 10/1
  In1/1 -> [B1]
  [B1] -> FOWT1/4(Blade Pitch(rad))
  [B1] -> FOWT2/4(Blade Pitch(rad))
  [B1] -> FOWT3/4(Blade Pitch(rad))
  [B1] -> FOWT4/4(Blade Pitch(rad))
  [B1] -> FOWT5/4(Blade Pitch(rad))
  [B1] -> FOWT6/4(Blade Pitch(rad))
